simulink model "compartment"  (R2020b)
settings: Solver=VariableStepAuto  StartTime=0.0  StopTime=30  RelTol=1e-3
values from neighbouring files (symbols this model uses):
  A = [-(Q+Qo)/V1 Q/V1 ... (first row only)    [compartment_script.m]
  B = [1/V1; 0]    [compartment_script.m]
libraries: simulink x1
settings Model: Creator=kjartan  LastModifiedBy=kjartan

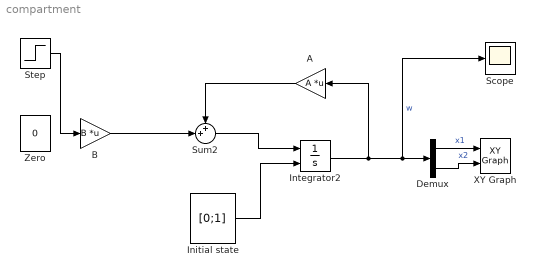
== system compartment ==
  A : Gain  Gain=A  Multiplication=Matrix(K*u) (u vector)
  B : Gain  Gain=B  Multiplication=Matrix(K*u)
  Demux : Demux  Outputs=2
  Initial state : Constant  Value=[0;1]
  Integrator2 : Integrator  InitialConditionSource=external
  Scope : Scope
  Step : Step  SampleTime=0
  Sum2 : Sum  Inputs=++|
  XY Graph : simulink/Sinks/XY Graph  xmin=0  xmax=2  ymin=0  ymax=2  st=-1
  Zero : Constant  Value=0  OutDataTypeStr=Inherit: Inherit via back propagation
  wires:
  Initial state/1 -> Integrator2/2
  B/1 -> Sum2/2
  Sum2/1 -> Integrator2/1
  Integrator2/1 -> Scope/1, Demux/1, A/1  "w"
  A/1 -> Sum2/1
  Demux/1 -> XY Graph/1  "x1"
  Demux/2 -> XY Graph/2  "x2"
  Step/1 -> B/1
